simulink model "demo"  (R2016b)
settings: Solver=FixedStepDiscrete  StartTime=0.0  StopTime=10.0  FixedStep=0.01  RelTol=1e-3
settings Model: Creator=jgillis  LastModifiedBy=jgillis

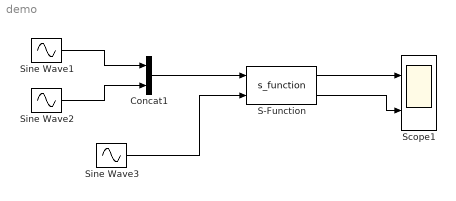
== system demo ==
  Concat1 : Concatenate
  S-Function : S-Function  FunctionName=s_function  SFunctionDeploymentMode=off  EnableBusSupport=off
  Scope1 : Scope  NumInputPorts=2
  Sine Wave1 : Sin  SampleTime=0
  Sine Wave2 : Sin  Phase=0.5  SampleTime=0
  Sine Wave3 : Sin  Frequency=3  SampleTime=0
  wires:
  S-Function/1 -> Scope1/1
  S-Function/2 -> Scope1/2
  Sine Wave1/1 -> Concat1/1
  Sine Wave2/1 -> Concat1/2
  Concat1/1 -> S-Function/1
  Sine Wave3/1 -> S-Function/2
